simulink model "modular_th"  (R2018b)
settings: Solver=ode15s  StartTime=0.0  StopTime=duration_s  MaxStep=5  RelTol=1e-3  AbsTol=1e-3
libraries: ayazController_cl x1, ayazGroundStation_cl x1, ayazLiftingBody_cl x1, ayazTethers_cl x1, ayazWinches_cl x1
settings Model: Creator=mcobb  LastModifiedBy=mcobb

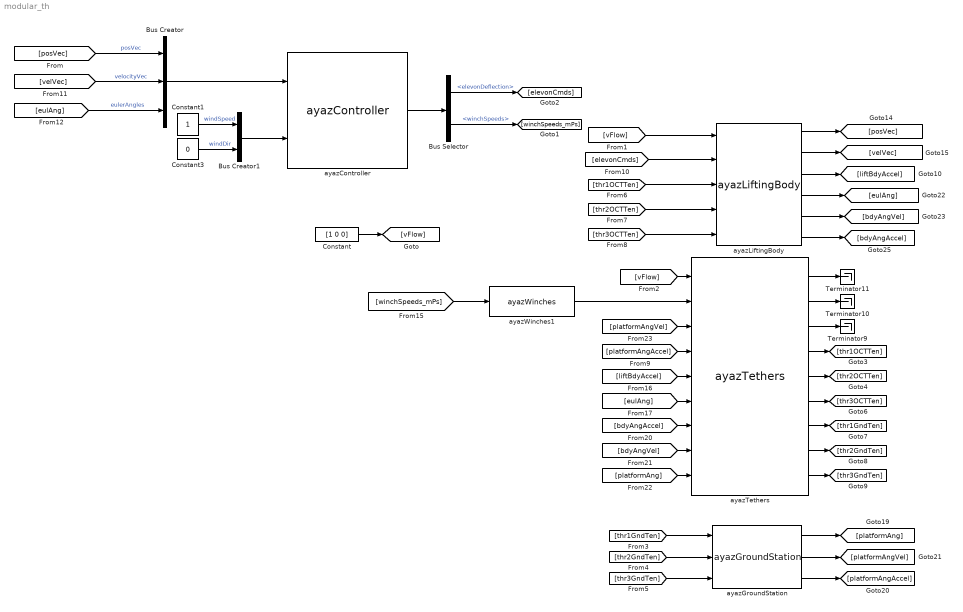
== system modular_th ==
  Bus Creator : BusCreator  Inputs=3  OutDataTypeStr=Bus: plantBus
  Bus Creator1 : BusCreator  Inputs=2  OutDataTypeStr=Bus: envBus
  Bus Selector : BusSelector  OutputSignals=elevonDeflection,winchSpeeds
  Constant : Constant  Value=[1 0 0]
  Constant1 : Constant
  Constant3 : Constant  Value=0
  Terminator10 : Terminator
  Terminator11 : Terminator
  Terminator9 : Terminator
  ayazController : ayazController_cl/ayazController  SystemSampleTime=-1  VariantControl=VSS_controller_ayazController
  ayazGroundStation : ayazGroundStation_cl/ayazGroundStation  SystemSampleTime=-1
  ayazLiftingBody : ayazLiftingBody_cl/ayazLiftingBody  SystemSampleTime=-1
  ayazTethers : ayazTethers_cl/ayazTethers  SystemSampleTime=-1
  ayazWinches1 : ayazWinches_cl/ayazWinches  SystemSampleTime=-1
  wires:
  Constant/1 -> [vFlow]
  ayazController/1 -> Bus Selector/1
  Bus Selector/2 -> [winchSpeeds_mPs]  "<winchSpeeds>"
  Bus Selector/1 -> [elevonCmds]  "<elevonDeflection>"
  Bus Creator/1 -> ayazController/1
  Bus Creator1/1 -> ayazController/2
  Constant1/1 -> Bus Creator1/1  "windSpeed"
  Constant3/1 -> Bus Creator1/2  "windDir"
  [posVec] -> Bus Creator/1  "posVec"
  [velVec] -> Bus Creator/2  "velocityVec"
  [eulAng] -> Bus Creator/3  "eulerAngles"
  [thr3GndTen] -> ayazGroundStation/3
  [elevonCmds] -> ayazLiftingBody/2
  ayazTethers/6 -> [thr3OCTTen]
  [vFlow] -> ayazLiftingBody/1
  [thr1GndTen] -> ayazGroundStation/1
  [vFlow] -> ayazTethers/1
  [thr3OCTTen] -> ayazLiftingBody/5
  ayazLiftingBody/2 -> [velVec]
  [winchSpeeds_mPs] -> ayazWinches1/1
  ayazTethers/3 -> Terminator9/1
  ayazTethers/8 -> [thr2GndTen]
  ayazTethers/9 -> [thr3GndTen]
  ayazLiftingBody/5 -> [bdyAngVel]
  ayazTethers/7 -> [thr1GndTen]
  [platformAngVel] -> ayazTethers/3
  [bdyAngVel] -> ayazTethers/8
  ayazLiftingBody/6 -> [bdyAngAccel]
  [bdyAngAccel] -> ayazTethers/7
  [liftBdyAccel] -> ayazTethers/5
  [eulAng] -> ayazTethers/6
  ayazTethers/1 -> Terminator11/1
  [platformAngAccel] -> ayazTethers/4
  ayazTethers/5 -> [thr2OCTTen]
  ayazGroundStation/2 -> [platformAngVel]
  ayazGroundStation/1 -> [platformAng]
  ayazLiftingBody/4 -> [eulAng]
  [thr2OCTTen] -> ayazLiftingBody/4
  ayazWinches1/1 -> ayazTethers/2
  ayazLiftingBody/3 -> [liftBdyAccel]
  [thr2GndTen] -> ayazGroundStation/2
  [thr1OCTTen] -> ayazLiftingBody/3
  ayazGroundStation/3 -> [platformAngAccel]
  ayazTethers/4 -> [thr1OCTTen]
  ayazLiftingBody/1 -> [posVec]
  [platformAng] -> ayazTethers/9
  ayazTethers/2 -> Terminator10/1
